simulink model "PMSM_SMO_SMC"  (R2022b)
settings: Solver=VariableStepAuto  StartTime=0.0  StopTime=4  FixedStep=1e-5  MaxStep=1E-5  RelTol=1e-4
values from neighbouring files (symbols this model uses):
  a_SMO = 0.6    [PMSM_SMO_SMC.m]
  Id_ref = 0    [PMSM_SMO_SMC.m]
  Ki_d = 100    [PMSM_SMO_SMC.m]
  Ki_q = 100    [PMSM_SMO_SMC.m]
  Kp_d = 0.1    [PMSM_SMO_SMC.m]
  Kp_q = 10    [PMSM_SMO_SMC.m]
  p = 4    [PMSM_SMO_SMC.m]
  Rs = 2.875    [PMSM_SMO_SMC.m]
  Ts = 1e-4    (= 0.0001)    [PMSM_SMO_SMC.m]
  Vdc = 310    [PMSM_SMO_SMC.m]
undefined symbols (not defined in the file or in its folder): sigbuilder_block
libraries: slpidlib x3, spsVoltageMeasurementLib x3, spsPermanentMagnetSynchronousMachineLib x2, mcbcontrolslib x2, spsAlphaBetaZerotodq0Lib x1, eeTransforms x1, spsDCVoltageSourceLib x1, spsTwoLevelConverterLib x1, spsThreePhaseVIMeasurementLib x1, spsSVPWMGenerator2LevelLib x1, spsdq0toAlphaBetaZeroLib x1, mcbsensorlessestimatorlib x1
settings Model: SimulationMode=accelerator  Creator=The MathWorks, Inc.  LastModifiedBy=DELL
settings DataIOCC: ExternalInput=[]  SaveFormat=Array  SaveOutput=off  SaveTime=off  ReturnWorkspaceOutputs=off  SignalLoggingName=sigsOut
settings OptimizationCC: BlockReduction=off  BooleanDataType=off  ExpressionDepthLimit=2147483647  InitFltsAndDblsToZero=on  EfficientMapNaN2IntZero=off  LifeSpan=inf
settings DebuggingCC: UnderspecifiedInitializationDetection=Classic  MergeDetectMultiDrivingBlocksExec=none  CheckExecutionContextPreStartOutputMsg=on  SignalResolutionControl=TryResolveAllWithWarning  MultiTaskDSMMsg=warning  MultiTaskCondExecSysMsg=none  SigSpecEnsureSampleTimeMsg=none  ParameterPrecisionLossMsg=none  FcnCallInpInsideContextMsg=warning  UnconnectedInputMsg=warning  UnconnectedOutputMsg=warning  UnconnectedLineMsg=warning  StateNameClashWarn=warning  SFUnexpectedBacktrackingDiag=warning  SFNoUnconditionalDefaultTransitionDiag=warning  SFExecutionAtInitializationDiag=none  SFMachineParentedDataDiag=warning  ArithmeticOperatorsInVariantConditions=warning
settings HardwareCC: ProdBitPerPointer=32  ProdBitPerSizeT=32  ProdBitPerPtrDiffT=32  ProdLargestAtomicFloat=None  ProdIntDivRoundTo=Undefined  ProdEndianess=Unspecified  ProdWordSize=32  ProdHWDeviceType=32-bit Generic  TargetUnknown=on
settings ModelReferenceCC: EnableRefExpFcnMdlSchedulingChecks=on  PropagateSignalLabelsOutOfModel=off
settings SFSimCC: SimUseLocalCustomCode=off  CustomCodeUndefinedFunction=UseInterfaceOnly
settings RTWCC: RTWUseLocalCustomCode=off
settings CodeAppCC: StateflowObjectComments=on
settings GRTTargetCC: TargetLangStandard=C89/C90 (ANSI)  CombineOutputUpdateFcns=off  GRTInterface=on
settings ConfigComp: CovMetricSettings=dw  CovSaveCumulativeToWorkspaceVar=on  CovSaveSingleToWorkspaceVar=on  CovExternalEMLEnable=off  CovSFcnEnable=off
settings SimscapeCC: SimscapeNormalizeSystem=off  SimscapeNominalValues={1, 'bar'; 1, 'cm^3/s'; 1, 'bar*kg/s'; 1, 'kJ/kg'; 1, 'kW'; }

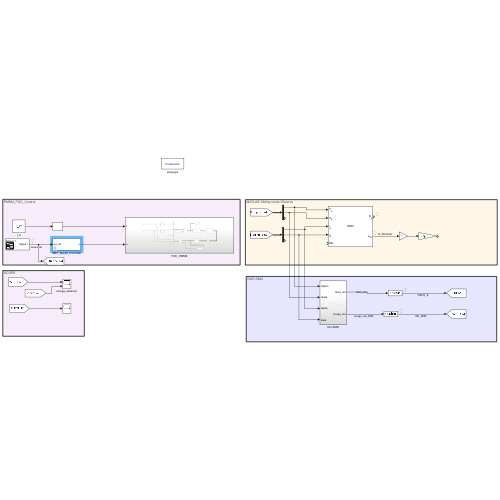
[thumbnail: Simulink's stored preview of the top-level diagram]
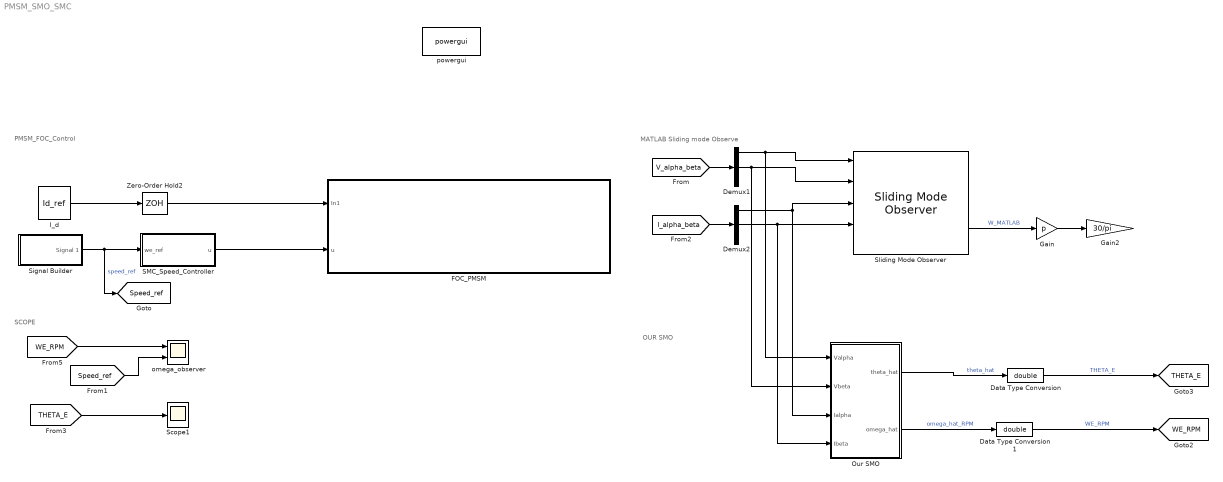
== system PMSM_SMO_SMC ==
  note: OUR SMO
  note: PMSM_FOC_Control
  note: MATLAB Sliding mode Observe
  note: SCOPE
  Data Type Conversion : DataTypeConversion  OutDataTypeStr=double  SaturateOnIntegerOverflow=off  RndMeth=Floor
  Data Type Conversion1 : DataTypeConversion  OutDataTypeStr=double  SaturateOnIntegerOverflow=off  RndMeth=Floor
  Demux1 : Demux  Outputs=3
  Demux2 : Demux  Outputs=3
  FOC_PMSM : Subsystem
  Gain : Gain  Gain=p
  Gain2 : Gain  Gain=30/pi  SaturateOnIntegerOverflow=on  OutDataTypeStr=Inherit: Same as input  ParamDataTypeStr=Inherit: Same as input
  I_d : Constant  Value=Id_ref
  Our SMO : Subsystem
  SMC_Speed_Controller : Subsystem  mask{TL=0.2, J=0.0008, B=0, p=4, lambda=0.175}
      mask prompts: TL "Torque Load"; J "Inetira"; B "Friction"; p "Pole"; lambda "flux linkage"
  Scope1 : Scope
  Signal Builder : Subsystem  Tag=STV Subsys  LoadFcn=sigbuilder_block('load');  StartFcn=sigbuilder_block('start');  StopFcn=sigbuilder_block('stop');  ClipboardFcn=sigbuilder_block('clipboard');  mask(Sigbuilder block){tuvar=[0:10]}
      mask help: Simulink:masks:SigbuilderBlock_MD
      mask init:
      | if ~strcmp(get_param(bdroot(gcbh),'SimulationStatus'),'stopped') tuvar = sigbuilder_block('maskInit'); end
      settings: CopyFcn=sigbuilder_block('copy');  DeleteFcn=sigbuilder_block('delete');  ModelCloseFcn=sigbuilder_block('modelClose');  PreSaveFcn=sigbuilder_block('preSave');  PauseFcn=sigbuilder_block('pause');  ContinueFcn=sigbuilder_block('continue');  NameChangeFcn=sigbuilder_block('namechange');  OpenFcn=sigbuilder_block('open',[437.6 199.2 550.4 400 ]);  CloseFcn=sigbuilder_block('close');
      mask Display: plot(0, 0, 100, 100,[2, 2, 32, 32, 2], [68, 8, 8, 68, 68],[32, 2], [38, 38], [32, 19, 2],[53, 60, 44], [32, 17, 17, 2],[16, 16, 31, 31]);txt = getActiveGroup(gcbh);text(2, 100, txt,'verticalAlignment', 'top');
  Sliding Mode Observer : mcbsensorlessestimatorlib/Sliding Mode Observer  InputUnit=SI unit  BlkSampleTime=1E-4  StatorResistance=StatorResistance  StatorInductance=StatorInductance  MaxApplicationSpeed=6000  PolePairs=PolePairs  MaxStatorVoltage=MaxStatorVoltage  MaxStatorCurrent=5  DisturbanceObserverGain=DisturbanceObserverGain  CurrentObserverGain=CurrentObserverGain  CutoffFreq=CutoffFreq  PositionUnit=Radians  PositionDataType=single  SpeedUnit=Radians/sec  PerUnitSpeed=6000  SpeedDataType=single
      settings: LibrarySourceBlock=mcblib/Sensorless Estimators/Sliding Mode Observer
  Zero-Order Hold2 : ZeroOrderHold  SampleTime=Ts
  omega_observer : Scope  NumInputPorts=2
  powergui : sps_lib/powergui  Priority=1  SimulationMode=Continuous  SampleTime=50e-6  frequency=60  Iterations=50  frequencyindice=0  Pbase=100e6  ErrMax=1e-4  UnitsV=kV  UnitsW=MW  buscounter=0  FunctionMessages=off  echomessages=off  EnableUseOfTLC=off  CurrentSourceSwitches=off  DisableSnubberDevices=off  DisableRonSwitches=off  DisableVfSwitches=off  DisplayEquations=off  AutomaticDiscreteSolvers=off  SolverType=Tustin/Backward Euler (TBE)  Interpol=off  ExternalGateDelay=off  methode=off  Ts=100  x0status=blocks  SPID=on  SwTol=0  HookPort=off  NonlinearTolerance=1e-4  nMaxIteration=100  ContinueOnMaxIteration=off  RestoreLinks=warning  ResistiveCurrentMeasurement=off  Frange=[0:2:500]  Ylog=off  Xlog=on  ShowGrid=off  save=off  variable=ZData  structure=0  ZoomFFT=off  StartTime=0.0  cycles=1  DisplayStyle=1  fundamental=60  FreqAxis=off  MaxFrequency=1000  frequencyindicesteady=1  RmsSteady=1  display=off
  tag scope: Speed_ref=global, THETA_E=global, WE_RPM=global
  wires:
  [V_alpha_beta] -> Demux1/1
  [I_alpha_beta] -> Demux2/1
  Gain/1 -> Gain2/1
  I_d/1 -> Zero-Order Hold2/1
  Zero-Order Hold2/1 -> FOC_PMSM/1(In1)
  Sliding Mode Observer/2 -> Gain/1  "W_MATLAB"
  Demux1/1 -> Our SMO/1(Valpha), Sliding Mode Observer/1
  Demux1/2 -> Our SMO/2(Vbeta), Sliding Mode Observer/2
  Demux2/1 -> Our SMO/3(Ialpha), Sliding Mode Observer/3
  Demux2/2 -> Our SMO/4(Ibeta), Sliding Mode Observer/4
  Our SMO/2(omega_hat) -> Data Type Conversion1/1  "omega_hat_RPM"
  Data Type Conversion/1 -> [THETA_E]  "THETA_E"
  Data Type Conversion1/1 -> [WE_RPM]  "WE_RPM"
  SMC_Speed_Controller/1(u) -> FOC_PMSM/2(u)
  Our SMO/1(theta_hat) -> Data Type Conversion/1  "theta_hat"
  Signal Builder/1(Signal 1) -> [Speed_ref], SMC_Speed_Controller/1(we_ref)  "speed_ref"
  [WE_RPM] -> omega_observer/1
  [THETA_E] -> Scope1/1
  [Speed_ref] -> omega_observer/2

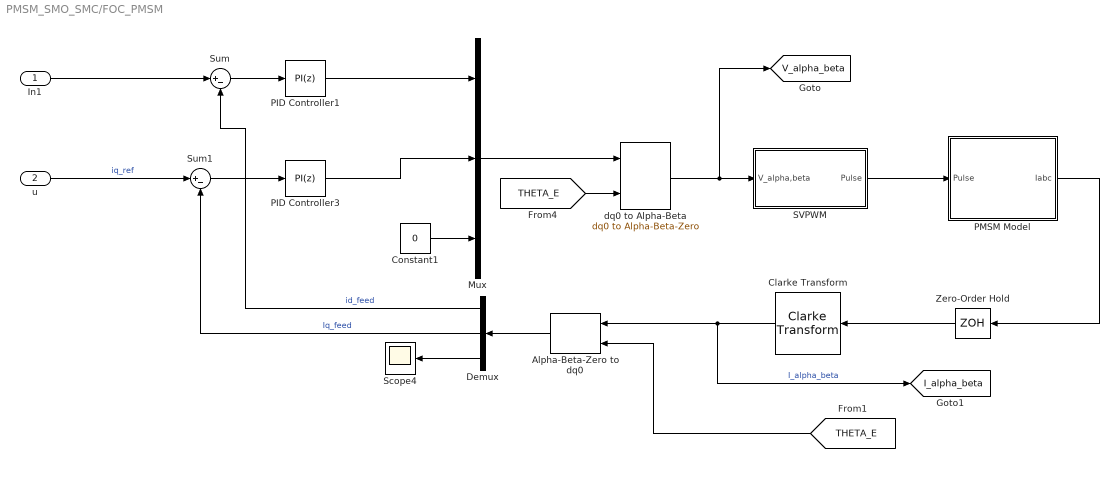
== system PMSM_SMO_SMC/FOC_PMSM ==
  In1 : Inport
  u : Inport  Port=2
  Alpha-Beta-Zero to dq0 : spsAlphaBetaZerotodq0Lib/Alpha-Beta-Zero to dq0  Alignment=Aligned with phase A axis
  Clarke Transform : eeTransforms/Clarke Transform  PowerInvariant=off
      settings: LibrarySourceBlock=|
      | ee_sl_lib/Mathematical
      | Transforms/Clarke Transform
  Constant1 : Constant  Value=0
  Demux : Demux  Outputs=3
  Mux : Mux  Inputs=3
  PID Controller1 : slpidlib/PID Controller  Controller=PI  Form=Parallel  TimeDomain=Discrete-time  UseExternalTs=off  SampleTime=1E-4  IntegratorMethod=Forward Euler  FilterMethod=Forward Euler  ControllerParametersSource=internal  P=Kp_d  I=Ki_d  UseKiTs=off  D=0  N=100  UseFilter=on  TunerSelectOption=Transfer Function Based (PID Tuner App)  InitialConditionSource=internal  InitialConditionForIntegrator=0  InitialConditionForFilter=0  DifferentiatorICPrevScaledInput=0  ExternalReset=none  TrackingMode=off  Kt=1  LimitOutput=off  SatLimitsSource=internal  UpperSaturationLimit=inf  LowerSaturationLimit=-inf  LinearizeAsGain=on  AntiWindupMode=none  Kb=1  LimitIntegrator=off  UpperIntegratorSaturationLimit=inf  LowerIntegratorSaturationLimit=-inf  POutMin=[]  POutMax=[]  IOutMin=[]  IOutMax=[]  DOutMin=[]  DOutMax=[]  NOutMin=[]  NOutMax=[]  SumOutMin=[]  SumOutMax=[]  SaturationOutMin=[]  SaturationOutMax=[]  PParamMin=[]  PParamMax=[]  IParamMin=[]  IParamMax=[]  DParamMin=[]  DParamMax=[]  NParamMin=[]  NParamMax=[]  KbParamMin=[]  KbParamMax=[]  KtParamMin=[]  KtParamMax=[]  KbOutMin=[]  KbOutMax=[]  KtOutMin=[]  KtOutMax=[]  IntegratorOutMin=[]  IntegratorOutMax=[]  FilterOutMin=[]  FilterOutMax=[]  SumI1OutMin=[]  SumI1OutMax=[]  SumI2OutMin=[]  SumI2OutMax=[]  SumI3OutMin=[]  SumI3OutMax=[]  SumI4OutMin=[]  SumI4OutMax=[]  SumDOutMin=[]  SumDOutMax=[]  DifferentiatorOutMin=[]  DifferentiatorOutMax=[]  FilterDiffOutCoefMin=[]  FilterDiffOutCoefMax=[]  ReciprocalOutMin=[]  ReciprocalOutMax=[]  SumDenOutMin=[]  SumDenOutMax=[]  SumNumOutMin=[]  SumNumOutMax=[]  DivideOutMin=[]  DivideOutMax=[]  UdiffTsProdOutMin=[]  UdiffTsProdOutMax=[]  NTsProdOutMin=[]  NTsProdOutMax=[]  UintegralTsProdOutMin=[]  UintegralTsProdOutMax=[]  UngainTsProdOutMin=[]  UngainTsProdOutMax=[]  ClampingZeroOutDataTypeStr=Inherit: Inherit via back propagation  ClampingZeroOutMin=[]  ClampingZeroOutMax=[]  FilterDenConstantOutDataTypeStr=Inherit: Inherit via back propagation  FilterDenConstantOutMin=[]  FilterDenConstantOutMax=[]  PCopyOutDataTypeStr=Inherit: Inherit via back propagation  PCopyOutMin=[]  PCopyOutMax=[]  NCopyOutDataTypeStr=Inherit: Inherit via back propagation  NCopyOutMin=[]  NCopyOutMax=[]  IntegratorContinuousStateAttributes=''  IntegratorStateMustResolveToSignalObject=off  IntegratorRTWStateStorageClass=Auto  FilterContinuousStateAttributes=''  FilterStateMustResolveToSignalObject=off  FilterRTWStateStorageClass=Auto  ParallelPVariant=InternalParameters  IdealPVariant=Disabled  IVariant=InternalParameters  DVariant=Disabled  IntegratorVariant=Discrete  SatVariant=Disabled  AWVariant=Passthrough  PCopyVariant=Disabled  TRVariant=Disabled  FdbkBlocksVariant=Forward  IdealPFdbkVariant=Disabled  SatFdbkVariant=Disabled  DerivativeFilterVariant=Disabled  NVariant=Disabled  NCopyVariant=Disabled_SignalSpec  FilterICVariant=Disabled  IntegratorICVariant=InternalICs  ExternalResetVariant=Disabled  TRSumVariant=Passthrough  SumFdbkVariant=Disabled  SumVariant=Sum_PI  TsampFilterVariant=InternalTs  TsampNgainVariant=Passthrough  TsampIntegralVariant=Passthrough  ExternalSaturationOutDataTypeStr=Inherit: Same as second input
  PID Controller3 : slpidlib/PID Controller  Controller=PI  Form=Parallel  TimeDomain=Discrete-time  UseExternalTs=off  SampleTime=1E-4  IntegratorMethod=Forward Euler  FilterMethod=Forward Euler  ControllerParametersSource=internal  P=Kp_q  I=Ki_q  UseKiTs=off  D=0  N=100  UseFilter=on  TunerSelectOption=Transfer Function Based (PID Tuner App)  InitialConditionSource=internal  InitialConditionForIntegrator=0  InitialConditionForFilter=0  DifferentiatorICPrevScaledInput=0  ExternalReset=none  TrackingMode=off  Kt=1  LimitOutput=off  SatLimitsSource=internal  UpperSaturationLimit=inf  LowerSaturationLimit=-inf  LinearizeAsGain=on  AntiWindupMode=none  Kb=1  LimitIntegrator=off  UpperIntegratorSaturationLimit=inf  LowerIntegratorSaturationLimit=-inf  POutMin=[]  POutMax=[]  IOutMin=[]  IOutMax=[]  DOutMin=[]  DOutMax=[]  NOutMin=[]  NOutMax=[]  SumOutMin=[]  SumOutMax=[]  SaturationOutMin=[]  SaturationOutMax=[]  PParamMin=[]  PParamMax=[]  IParamMin=[]  IParamMax=[]  DParamMin=[]  DParamMax=[]  NParamMin=[]  NParamMax=[]  KbParamMin=[]  KbParamMax=[]  KtParamMin=[]  KtParamMax=[]  KbOutMin=[]  KbOutMax=[]  KtOutMin=[]  KtOutMax=[]  IntegratorOutMin=[]  IntegratorOutMax=[]  FilterOutMin=[]  FilterOutMax=[]  SumI1OutMin=[]  SumI1OutMax=[]  SumI2OutMin=[]  SumI2OutMax=[]  SumI3OutMin=[]  SumI3OutMax=[]  SumI4OutMin=[]  SumI4OutMax=[]  SumDOutMin=[]  SumDOutMax=[]  DifferentiatorOutMin=[]  DifferentiatorOutMax=[]  FilterDiffOutCoefMin=[]  FilterDiffOutCoefMax=[]  ReciprocalOutMin=[]  ReciprocalOutMax=[]  SumDenOutMin=[]  SumDenOutMax=[]  SumNumOutMin=[]  SumNumOutMax=[]  DivideOutMin=[]  DivideOutMax=[]  UdiffTsProdOutMin=[]  UdiffTsProdOutMax=[]  NTsProdOutMin=[]  NTsProdOutMax=[]  UintegralTsProdOutMin=[]  UintegralTsProdOutMax=[]  UngainTsProdOutMin=[]  UngainTsProdOutMax=[]  ClampingZeroOutDataTypeStr=Inherit: Inherit via back propagation  ClampingZeroOutMin=[]  ClampingZeroOutMax=[]  FilterDenConstantOutDataTypeStr=Inherit: Inherit via back propagation  FilterDenConstantOutMin=[]  FilterDenConstantOutMax=[]  PCopyOutDataTypeStr=Inherit: Inherit via back propagation  PCopyOutMin=[]  PCopyOutMax=[]  NCopyOutDataTypeStr=Inherit: Inherit via back propagation  NCopyOutMin=[]  NCopyOutMax=[]  IntegratorContinuousStateAttributes=''  IntegratorStateMustResolveToSignalObject=off  IntegratorRTWStateStorageClass=Auto  FilterContinuousStateAttributes=''  FilterStateMustResolveToSignalObject=off  FilterRTWStateStorageClass=Auto  ParallelPVariant=InternalParameters  IdealPVariant=Disabled  IVariant=InternalParameters  DVariant=Disabled  IntegratorVariant=Discrete  SatVariant=Disabled  AWVariant=Passthrough  PCopyVariant=Disabled  TRVariant=Disabled  FdbkBlocksVariant=Forward  IdealPFdbkVariant=Disabled  SatFdbkVariant=Disabled  DerivativeFilterVariant=Disabled  NVariant=Disabled  NCopyVariant=Disabled_SignalSpec  FilterICVariant=Disabled  IntegratorICVariant=InternalICs  ExternalResetVariant=Disabled  TRSumVariant=Passthrough  SumFdbkVariant=Disabled  SumVariant=Sum_PI  TsampFilterVariant=InternalTs  TsampNgainVariant=Passthrough  TsampIntegralVariant=Passthrough  ExternalSaturationOutDataTypeStr=Inherit: Same as second input
  PMSM Model : Subsystem
  SVPWM : Subsystem
  Scope4 : Scope
  Sum : Sum  Inputs=|+-
  Sum1 : Sum  Inputs=|+-
  Zero-Order Hold : ZeroOrderHold  SampleTime=Ts
  dq0 to Alpha-Beta : spsdq0toAlphaBetaZeroLib/dq0 to Alpha-Beta-Zero  Alignment=Aligned with phase A axis
  tag scope: I_alpha_beta=global, V_alpha_beta=global
  wires:
  [THETA_E] -> Alpha-Beta-Zero to dq0/2
  Clarke Transform/1 -> [I_alpha_beta], Alpha-Beta-Zero to dq0/1  "I_alpha_beta"
  PMSM Model/1(Iabc) -> Zero-Order Hold/1
  Mux/1 -> dq0 to Alpha-Beta/1
  u/1 -> Sum1/1  "iq_ref"
  Sum1/1 -> PID Controller3/1
  SVPWM/1(Pulse) -> PMSM Model/1(Pulse)
  dq0 to Alpha-Beta/1 -> [V_alpha_beta], SVPWM/1(V_alpha,beta)
  Demux/1 -> Sum/2  "id_feed"
  Constant1/1 -> Mux/3
  Demux/3 -> Scope4/1
  [THETA_E] -> dq0 to Alpha-Beta/2
  Sum/1 -> PID Controller1/1
  Demux/2 -> Sum1/2  "Iq_feed"
  Alpha-Beta-Zero to dq0/1 -> Demux/1
  In1/1 -> Sum/1
  Zero-Order Hold/1 -> Clarke Transform/1
  PID Controller1/1 -> Mux/1
  PID Controller3/1 -> Mux/2

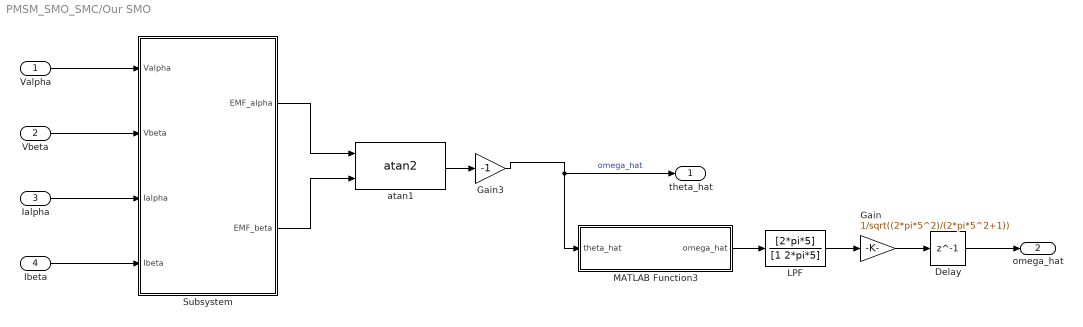
== system PMSM_SMO_SMC/Our SMO ==
  Valpha : Inport
  Vbeta : Inport  Port=2
  Ialpha : Inport  Port=3
  Ibeta : Inport  Port=4
  Delay : Delay  DelayLength=1
  Gain : Gain  Gain=1/sqrt((2*pi*5^2)/(2*pi*5^2+1))
  Gain3 : Gain  Gain=-1
  LPF : TransferFcn  Numerator=[2*pi*5]  Denominator=[1 2*pi*5]
  MATLAB Function3 : MATLAB Function  TreatAsAtomicUnit=on
  Subsystem : Subsystem
  atan1 : mcbcontrolslib/atan2  outputUnit=Radians
  theta_hat : Outport
  omega_hat : Outport  Port=2
  wires:
  Valpha/1 -> Subsystem/1(Valpha)
  Vbeta/1 -> Subsystem/2(Vbeta)
  Ialpha/1 -> Subsystem/3(Ialpha)
  Ibeta/1 -> Subsystem/4(Ibeta)
  atan1/1 -> Gain3/1
  MATLAB Function3/1(omega_hat) -> LPF/1
  LPF/1 -> Gain/1
  Gain3/1 -> theta_hat/1, MATLAB Function3/1(theta_hat)  "omega_hat"
  Subsystem/1(EMF_alpha) -> atan1/1
  Subsystem/2(EMF_beta) -> atan1/2
  Delay/1 -> omega_hat/1
  Gain/1 -> Delay/1

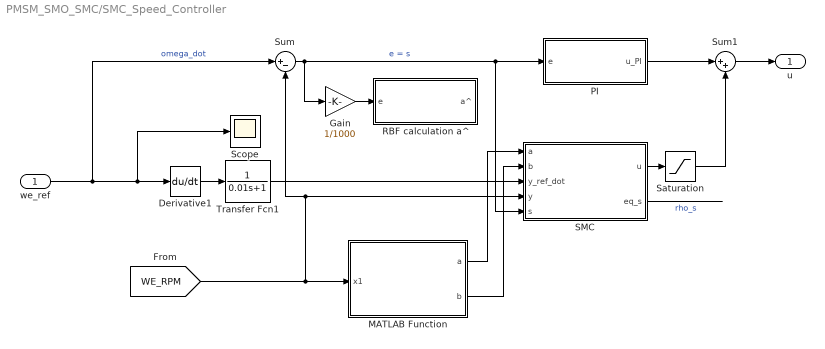
== system PMSM_SMO_SMC/SMC_Speed_Controller ==
  we_ref : Inport
  Derivative1 : Derivative
  Gain : Gain  Gain=1/1000
  MATLAB Function : MATLAB Function  TreatAsAtomicUnit=on
  PI : Subsystem
  RBF calculation a^ : Subsystem
  SMC : MATLAB Function  TreatAsAtomicUnit=on
  Saturation : Saturate  UpperLimit=3  LowerLimit=-3
  Scope : Scope
  Sum : Sum  Inputs=|+-
  Sum1 : Sum  Inputs=|++
  Transfer Fcn1 : TransferFcn  Denominator=[0.01 1]
  u : Outport
  wires:
  [WE_RPM] -> Sum/2, SMC/4(y), MATLAB Function/1(x1)
  we_ref/1 -> Derivative1/1, Scope/1, Sum/1  "omega_dot"
  MATLAB Function/2(b) -> SMC/2(b)
  Sum/1 -> Gain/1, PI/1(e), SMC/5(s)  "e = s"
  SMC/1(u) -> Saturation/1
  SMC/2(eq_s) -> ?  "rho_s"
  Gain/1 -> RBF calculation a^/1(e)
  MATLAB Function/1(a) -> SMC/1(a)
  Derivative1/1 -> Transfer Fcn1/1
  Transfer Fcn1/1 -> SMC/3(y_ref_dot)
  PI/1(u_PI) -> Sum1/1
  Saturation/1 -> Sum1/2
  Sum1/1 -> u/1

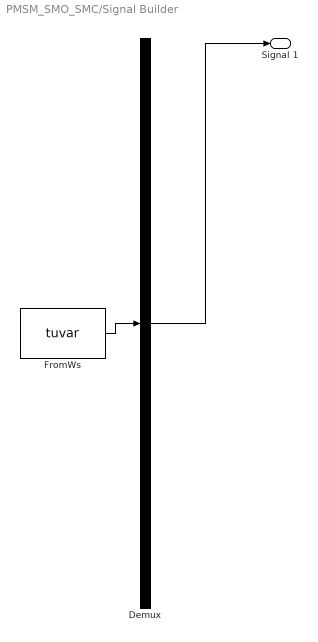
== system PMSM_SMO_SMC/Signal Builder ==
  Demux : Demux  Tag=STV Demux  Outputs=1
      settings: DisplayOption=none
  FromWs : FromWorkspace  Tag=STV FromWs  VariableName=tuvar
      SigBuilderData=|
      | common.afterFinalStr = 'Extrapolate'
      | common.sampleTime = 0
      | dataSet.timeRange = [0 10]
      | dataSet.name = 'Group 1'
      | sbobj.Groups.Name = 'Group 1'
      | sbobj.Groups.Signals.Name = 'Signal 1'
      | sbobj.Groups.Signals.XData = [0 4 4 6 6 8.04 8.04 10]
      | sbobj.Groups.Signals.YData = [1000 1000 200 200 1000 1000 600 600]
  Signal 1 : Outport  Tag=STV Outport
  wires:
  Demux/1 -> Signal 1/1
  FromWs/1 -> Demux/1

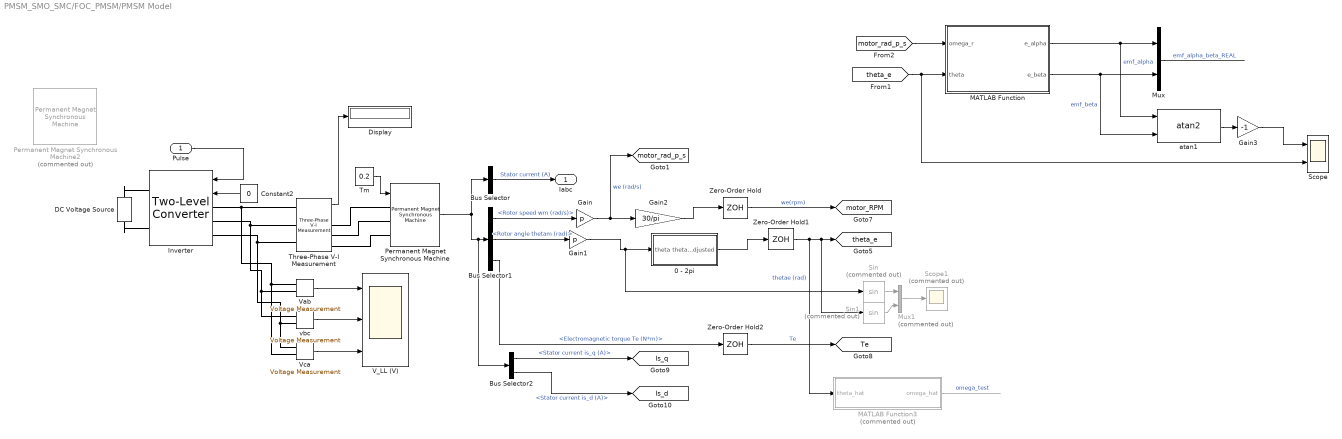
== system PMSM_SMO_SMC/FOC_PMSM/PMSM Model ==
  Pulse : Inport
  0 - 2pi : MATLAB Function  TreatAsAtomicUnit=on
  Bus Selector : BusSelector  OutputSignals=Stator current is_a (A),Stator current is_b (A),Stator current is_c (A)  OutputAsBus=on
  Bus Selector1 : BusSelector  OutputSignals=Rotor speed wm (rad/s),Rotor angle thetam (rad),Electromagnetic torque Te (N*m)
  Bus Selector2 : BusSelector  OutputSignals=Stator current is_q (A),Stator current is_d (A)
  Constant2 : Constant  Value=0
  "DC Voltage Source  " : spsDCVoltageSourceLib/DC Voltage Source  Amplitude=Vdc  Measurements=Voltage
  Display : Display
  Gain : Gain  Gain=p  SaturateOnIntegerOverflow=on  OutDataTypeStr=Inherit: Same as input  ParamDataTypeStr=Inherit: Same as input
  Gain1 : Gain  Gain=p  SaturateOnIntegerOverflow=on  OutDataTypeStr=Inherit: Same as input  ParamDataTypeStr=Inherit: Same as input
  Gain2 : Gain  Gain=30/pi  SaturateOnIntegerOverflow=on  OutDataTypeStr=Inherit: Same as input  ParamDataTypeStr=Inherit: Same as input
  Gain3 : Gain  Gain=-1
  Inverter : spsTwoLevelConverterLib/Two-Level Converter  ModelType=Switching devices  Ron=1e-3  Rs=1e6  Cs=inf  Vforward=[0,0]  Ron_Diode=1e-3  Rs_Diode=1e6  Cs_Diode=inf  Vf_Diode=1e-3  Rs_CurrentSource=inf  Ron_ACsource=1e-3
      settings: LibrarySourceBlock=sps_lib/Power Electronics/Two-Level Converter
  MATLAB Function : MATLAB Function  TreatAsAtomicUnit=on
  MATLAB Function3 : MATLAB Function  Commented=on  TreatAsAtomicUnit=on
  Mux : Mux  Inputs=2
  Mux1 : Mux  Commented=on  Inputs=2
  Permanent Magnet Synchronous Machine : spsPermanentMagnetSynchronousMachineLib/Permanent Magnet Synchronous Machine  NbPhases=3  FluxDistribution=Sinusoidal  RotorType=Round  MechanicalLoad=Torque Tm  PresetModel=No  ShowDetailedParameters=on  MeasurementBus=off  Resistance=Rs  Inductance=8.5e-3  dqInductances=[8.5e-3,8.5e-3]  La=Ls  MachineConstant=Flux linkage established by magnets (V.s)  Flux=lambda  VoltageCst=126.966  TorqueCst=1.05  Flat=120  Mechanical=[0.0008 1.349e-05 p 0]  PolePairs=4  InitialConditions=[0,0,0,0]  InitialConditions5ph=[0 0 0 0 0 0]  RefAngle=Aligned with phase A axis (original Park)  IterativeDiscreteModel=Trapezoidal non iterative  TsBlock=-1  TsPowergui=0
  Permanent Magnet Synchronous Machine2 : spsPermanentMagnetSynchronousMachineLib/Permanent Magnet Synchronous Machine  Commented=on  NbPhases=3  FluxDistribution=Sinusoidal  RotorType=Round  MechanicalLoad=Torque Tm  PresetModel=No  ShowDetailedParameters=on  MeasurementBus=off  Resistance=2.87  Inductance=8.5e-3  dqInductances=[8.5e-3,8.5e-3]  La=8.5*1e-3  MachineConstant=Flux linkage established by magnets (V.s)  Flux=0.175  VoltageCst=63.483  TorqueCst=0.525  Flat=120  Mechanical=[0.0008 1.349e-05 2 0]  PolePairs=2  InitialConditions=[0,0,0,0]  InitialConditions5ph=[0 0 0 0 0 0]  RefAngle=Aligned with phase A axis (original Park)  IterativeDiscreteModel=Trapezoidal non iterative  TsBlock=-1  TsPowergui=0
  Scope : Scope  NumInputPorts=2
  Scope1 : Scope  Commented=on
  Sin : Trigonometry  Commented=on
  Sin1 : Trigonometry  Commented=on
  Three-Phase V-I Measurement : spsThreePhaseVIMeasurementLib/Three-Phase V-I Measurement  VoltageMeasurement=phase-to-phase  SetLabelV=off  LabelV=Vabc  Vpu=off  VpuLL=off  CurrentMeasurement=yes  SetLabelI=off  LabelI=Iabc  Ipu=off  Pbase=100e6  Vbase=500e3  OutputType=Complex  PhasorSimulation=off  PSBequivalent=0
  Tm : Constant  Value=0.2
  V_LL (V) : Scope  NumInputPorts=3
  Vab : spsVoltageMeasurementLib/Voltage Measurement  Tag=PoWeRsYsTeMmEaSuReMeNt  PhasorSimulation=off  OutputType=Magnitude  PSBequivalent=0
  Vca : spsVoltageMeasurementLib/Voltage Measurement  Tag=PoWeRsYsTeMmEaSuReMeNt  PhasorSimulation=off  OutputType=Magnitude  PSBequivalent=0
  Zero-Order Hold : ZeroOrderHold  SampleTime=Ts
  Zero-Order Hold1 : ZeroOrderHold  SampleTime=Ts
  Zero-Order Hold2 : ZeroOrderHold  SampleTime=Ts
  atan1 : mcbcontrolslib/atan2  outputUnit=Radians
  vbc : spsVoltageMeasurementLib/Voltage Measurement  Tag=PoWeRsYsTeMmEaSuReMeNt  PhasorSimulation=off  OutputType=Magnitude  PSBequivalent=0
  Iabc : Outport
  tag scope: Is_d=global, Is_q=global, Te=global, motor_RPM=global, motor_rad_p_s=global, theta_e=global
  wires:
  Bus Selector1/1 -> Gain/1  "<Rotor speed wm (rad/s)>"
  Gain/1 -> [motor_rad_p_s], Gain2/1  "we (rad/s)"
  Permanent Magnet Synchronous Machine/1 -> Bus Selector/1, Bus Selector2/1, Bus Selector1/1
  Bus Selector1/2 -> Gain1/1  "<Rotor angle thetam (rad)>"
  Gain2/1 -> Zero-Order Hold/1
  Bus Selector/1 -> Iabc/1  "Stator current (A)"
  Bus Selector2/1 -> [Is_q]  "<Stator current is_q (A)>"
  Bus Selector1/3 -> Zero-Order Hold2/1  "<Electromagnetic torque Te (N*m)>"
  Bus Selector2/2 -> [Is_d]  "<Stator current is_d (A)>"
  Tm/1 -> Permanent Magnet Synchronous Machine/1
  vbc/1 -> V_LL (V)/2
  Vca/1 -> V_LL (V)/3
  Vab/1 -> V_LL (V)/1
  Pulse/1 -> Inverter/1
  Constant2/1 -> Inverter/2
  Zero-Order Hold/1 -> [motor_RPM]  "we(rpm)"
  Zero-Order Hold1/1 -> MATLAB Function3/1(theta_hat), Sin1/1, [theta_e]  "thetae (rad)"
  Zero-Order Hold2/1 -> [Te]  "Te"
  Three-Phase V-I Measurement/1 -> Display/1
  0 - 2pi/1(theta_adjusted) -> Zero-Order Hold1/1
  [motor_rad_p_s] -> MATLAB Function/1(omega_r)
  [theta_e] -> Scope/2, MATLAB Function/2(theta)
  MATLAB Function/1(e_alpha) -> atan1/1, Mux/1  "emf_alpha"
  MATLAB Function/2(e_beta) -> atan1/2, Mux/2  "emf_beta"
  Mux/1 -> ?  "emf_alpha_beta_REAL"
  atan1/1 -> Gain3/1
  Gain3/1 -> Scope/1
  MATLAB Function3/1(omega_hat) -> ?  "omega_test"
  Gain1/1 -> Sin/1, 0 - 2pi/1(theta)
  Sin/1 -> Mux1/1
  Sin1/1 -> Mux1/2
  Mux1/1 -> Scope1/1
  connections:
  vbc/LConn1 -- Inverter/LConn2 -- Three-Phase V-I Measurement/LConn2 -- Vab/LConn2
  vbc/LConn2 -- Inverter/LConn3 -- Three-Phase V-I Measurement/LConn3 -- Vca/LConn1
  Vab/LConn1 -- Three-Phase V-I Measurement/LConn1 -- Inverter/LConn1 -- Vca/LConn2
  "DC Voltage Source  "/RConn1 -- Inverter/RConn1
  "DC Voltage Source  "/LConn1 -- Inverter/RConn2
  Three-Phase V-I Measurement/RConn1 -- Permanent Magnet Synchronous Machine/LConn1
  Three-Phase V-I Measurement/RConn2 -- Permanent Magnet Synchronous Machine/LConn2
  Three-Phase V-I Measurement/RConn3 -- Permanent Magnet Synchronous Machine/LConn3

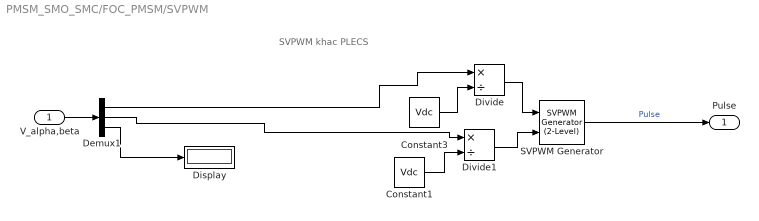
== system PMSM_SMO_SMC/FOC_PMSM/SVPWM ==
  note: SVPWM khac PLECS
  V_alpha,beta : Inport
  Constant1 : Constant  Value=Vdc
  Constant3 : Constant  Value=Vdc
  Demux1 : Demux  Outputs=3
  Display : Display
  Divide : Product  Inputs=*/
  Divide1 : Product  Inputs=*/
  SVPWM Generator : spsSVPWMGenerator2LevelLib/SVPWM Generator (2-Level)  InputType=alpha-beta components  SwitchingPattern=Pattern #1  Fc=10000  ParUref=[0.8 -30 50]  Ts=0
  Pulse : Outport
  wires:
  Demux1/2 -> Divide1/1
  Demux1/3 -> Display/1
  Demux1/1 -> Divide/1
  Divide/1 -> SVPWM Generator/1
  V_alpha,beta/1 -> Demux1/1
  Constant3/1 -> Divide/2
  SVPWM Generator/1 -> Pulse/1  "Pulse"
  Constant1/1 -> Divide1/2
  Divide1/1 -> SVPWM Generator/2

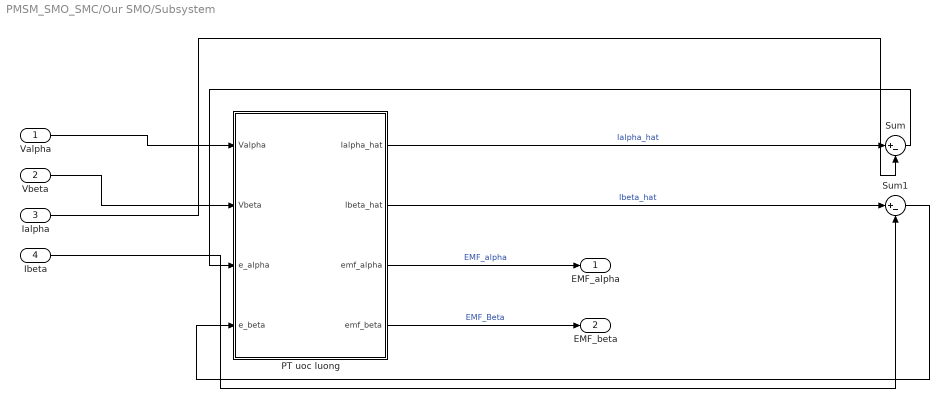
== system PMSM_SMO_SMC/Our SMO/Subsystem ==
  Valpha : Inport
  Vbeta : Inport  Port=2
  Ialpha : Inport  Port=3
  Ibeta : Inport  Port=4
  PT uoc luong : Subsystem
  Sum : Sum  Inputs=|+-
  Sum1 : Sum  Inputs=|+-
  EMF_alpha : Outport
  EMF_beta : Outport  Port=2
  wires:
  PT uoc luong/2(Ibeta_hat) -> Sum1/1  "Ibeta_hat"
  Sum1/1 -> PT uoc luong/4(e_beta)
  PT uoc luong/1(Ialpha_hat) -> Sum/1  "Ialpha_hat"
  Ibeta/1 -> Sum1/2
  Ialpha/1 -> Sum/2
  Sum/1 -> PT uoc luong/3(e_alpha)
  Valpha/1 -> PT uoc luong/1(Valpha)
  Vbeta/1 -> PT uoc luong/2(Vbeta)
  PT uoc luong/3(emf_alpha) -> EMF_alpha/1  "EMF_alpha"
  PT uoc luong/4(emf_beta) -> EMF_beta/1  "EMF_Beta"

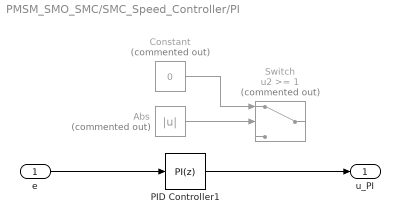
== system PMSM_SMO_SMC/SMC_Speed_Controller/PI ==
  e : Inport
  Abs : Abs  Commented=on  SaturateOnIntegerOverflow=off
  Constant : Constant  Commented=on  Value=0
  PID Controller1 : slpidlib/PID Controller  Controller=PI  Form=Parallel  TimeDomain=Discrete-time  UseExternalTs=off  SampleTime=1E-4  IntegratorMethod=Forward Euler  FilterMethod=Forward Euler  ControllerParametersSource=internal  P=0  I=0.1  UseKiTs=off  D=0  N=100  UseFilter=on  TunerSelectOption=Transfer Function Based (PID Tuner App)  InitialConditionSource=internal  InitialConditionForIntegrator=0  InitialConditionForFilter=0  DifferentiatorICPrevScaledInput=0  ExternalReset=none  TrackingMode=off  Kt=1  LimitOutput=off  SatLimitsSource=internal  UpperSaturationLimit=inf  LowerSaturationLimit=-inf  LinearizeAsGain=on  AntiWindupMode=none  Kb=1  LimitIntegrator=off  UpperIntegratorSaturationLimit=inf  LowerIntegratorSaturationLimit=-inf  POutMin=[]  POutMax=[]  IOutMin=[]  IOutMax=[]  DOutMin=[]  DOutMax=[]  NOutMin=[]  NOutMax=[]  SumOutMin=[]  SumOutMax=[]  SaturationOutMin=[]  SaturationOutMax=[]  PParamMin=[]  PParamMax=[]  IParamMin=[]  IParamMax=[]  DParamMin=[]  DParamMax=[]  NParamMin=[]  NParamMax=[]  KbParamMin=[]  KbParamMax=[]  KtParamMin=[]  KtParamMax=[]  KbOutMin=[]  KbOutMax=[]  KtOutMin=[]  KtOutMax=[]  IntegratorOutMin=[]  IntegratorOutMax=[]  FilterOutMin=[]  FilterOutMax=[]  SumI1OutMin=[]  SumI1OutMax=[]  SumI2OutMin=[]  SumI2OutMax=[]  SumI3OutMin=[]  SumI3OutMax=[]  SumI4OutMin=[]  SumI4OutMax=[]  SumDOutMin=[]  SumDOutMax=[]  DifferentiatorOutMin=[]  DifferentiatorOutMax=[]  FilterDiffOutCoefMin=[]  FilterDiffOutCoefMax=[]  ReciprocalOutMin=[]  ReciprocalOutMax=[]  SumDenOutMin=[]  SumDenOutMax=[]  SumNumOutMin=[]  SumNumOutMax=[]  DivideOutMin=[]  DivideOutMax=[]  UdiffTsProdOutMin=[]  UdiffTsProdOutMax=[]  NTsProdOutMin=[]  NTsProdOutMax=[]  UintegralTsProdOutMin=[]  UintegralTsProdOutMax=[]  UngainTsProdOutMin=[]  UngainTsProdOutMax=[]  ClampingZeroOutDataTypeStr=Inherit: Inherit via back propagation  ClampingZeroOutMin=[]  ClampingZeroOutMax=[]  FilterDenConstantOutDataTypeStr=Inherit: Inherit via back propagation  FilterDenConstantOutMin=[]  FilterDenConstantOutMax=[]  PCopyOutDataTypeStr=Inherit: Inherit via back propagation  PCopyOutMin=[]  PCopyOutMax=[]  NCopyOutDataTypeStr=Inherit: Inherit via back propagation  NCopyOutMin=[]  NCopyOutMax=[]  IntegratorContinuousStateAttributes=''  IntegratorStateMustResolveToSignalObject=off  IntegratorRTWStateStorageClass=Auto  FilterContinuousStateAttributes=''  FilterStateMustResolveToSignalObject=off  FilterRTWStateStorageClass=Auto  ParallelPVariant=InternalParameters  IdealPVariant=Disabled  IVariant=InternalParameters  DVariant=Disabled  IntegratorVariant=Discrete  SatVariant=Disabled  AWVariant=Passthrough  PCopyVariant=Disabled  TRVariant=Disabled  FdbkBlocksVariant=Forward  IdealPFdbkVariant=Disabled  SatFdbkVariant=Disabled  DerivativeFilterVariant=Disabled  NVariant=Disabled  NCopyVariant=Disabled_SignalSpec  FilterICVariant=Disabled  IntegratorICVariant=InternalICs  ExternalResetVariant=Disabled  TRSumVariant=Passthrough  SumFdbkVariant=Disabled  SumVariant=Sum_PI  TsampFilterVariant=InternalTs  TsampNgainVariant=Passthrough  TsampIntegralVariant=Passthrough  ExternalSaturationOutDataTypeStr=Inherit: Same as second input
  Switch : Switch  Commented=on  Threshold=1  SaturateOnIntegerOverflow=off  InputSameDT=off
  u_PI : Outport
  wires:
  e/1 -> PID Controller1/1
  PID Controller1/1 -> u_PI/1
  Constant/1 -> Switch/1
  Abs/1 -> Switch/2
  ? -> Abs/1

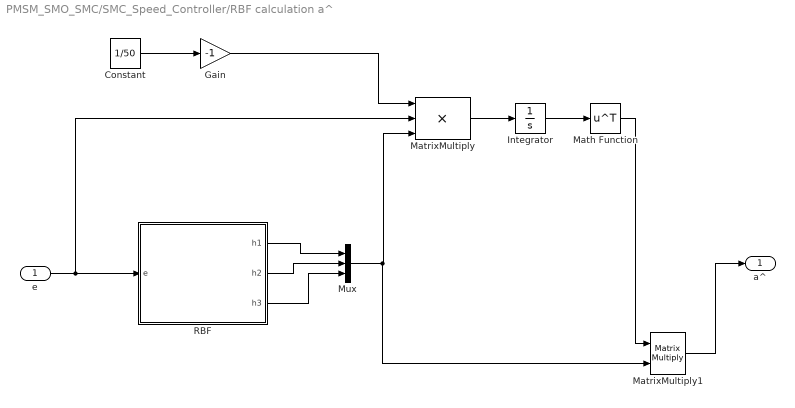
== system PMSM_SMO_SMC/SMC_Speed_Controller/RBF calculation a^ ==
  e : Inport
  Constant : Constant  Value=1/50
  Gain : Gain  Gain=-1
  Integrator : Integrator
  Math Function : Math  Operator=transpose
  MatrixMultiply : Product  Inputs=3
  MatrixMultiply1 : Product  Multiplication=Matrix(*)
  Mux : Mux  Inputs=3
  RBF : MATLAB Function  TreatAsAtomicUnit=on
  a^ : Outport
  wires:
  e/1 -> MatrixMultiply/2, RBF/1(e)
  RBF/1(h1) -> Mux/1
  RBF/2(h2) -> Mux/2
  RBF/3(h3) -> Mux/3
  Mux/1 -> MatrixMultiply1/2, MatrixMultiply/3
  Constant/1 -> Gain/1
  Gain/1 -> MatrixMultiply/1
  MatrixMultiply/1 -> Integrator/1
  Integrator/1 -> Math Function/1
  Math Function/1 -> MatrixMultiply1/1
  MatrixMultiply1/1 -> a^/1

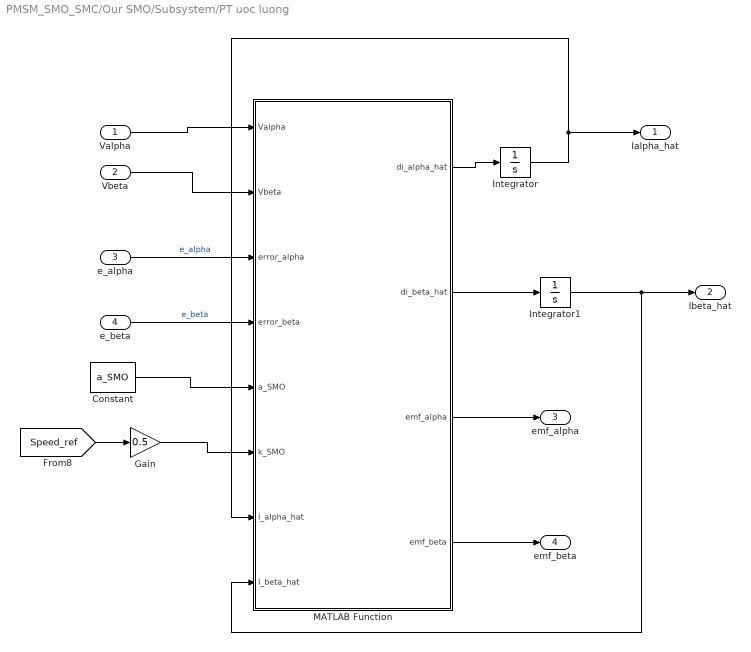
== system PMSM_SMO_SMC/Our SMO/Subsystem/PT uoc luong ==
  Valpha : Inport
  Vbeta : Inport  Port=2
  e_alpha : Inport  Port=3
  e_beta : Inport  Port=4
  Constant : Constant  Value=a_SMO
  Gain : Gain  Gain=0.5
  Integrator : Integrator
  Integrator1 : Integrator
  MATLAB Function : MATLAB Function  TreatAsAtomicUnit=on
  Ialpha_hat : Outport
  Ibeta_hat : Outport  Port=2
  emf_alpha : Outport  Port=3
  emf_beta : Outport  Port=4
  wires:
  Valpha/1 -> MATLAB Function/1(Valpha)
  Vbeta/1 -> MATLAB Function/2(Vbeta)
  e_alpha/1 -> MATLAB Function/3(error_alpha)  "e_alpha"
  e_beta/1 -> MATLAB Function/4(error_beta)  "e_beta"
  MATLAB Function/1(di_alpha_hat) -> Integrator/1
  MATLAB Function/2(di_beta_hat) -> Integrator1/1
  Integrator/1 -> MATLAB Function/7(I_alpha_hat), Ialpha_hat/1
  Integrator1/1 -> Ibeta_hat/1, MATLAB Function/8(I_beta_hat)
  MATLAB Function/4(emf_beta) -> emf_beta/1
  MATLAB Function/3(emf_alpha) -> emf_alpha/1
  Constant/1 -> MATLAB Function/5(a_SMO)
  Gain/1 -> MATLAB Function/6(k_SMO)
  [Speed_ref] -> Gain/1

== matlab function PMSM_SMO_SMC/Our SMO/Subsystem/PT uoc luong/MATLAB Function ==
  settings: updateMethod=DISCRETE  sampleTime=1E-4
  data: Valpha input; di_alpha_hat output; Vbeta input; error_alpha input; error_beta input; di_beta_hat output; emf_alpha output; emf_beta output; a_SMO input; k_SMO input; I_alpha_hat input; I_beta_hat input
function [di_alpha_hat, di_beta_hat, emf_alpha, emf_beta] = SMO_Observer(Valpha, Vbeta, error_alpha, error_beta, a_SMO,k_SMO, I_alpha_hat, I_beta_hat)
    Rs = 2.875; %Stator Resistance
    Ls = 8.5e-3; %Stator Inductance
    k = k_SMO ;
    a = a_SMO ;

    % Tính toán H_alpha và H_beta
    H_alpha = (2./(1 + exp(-a * error_alpha/20))) - 1;
    H_beta = (2./(1 + exp(-a * error_beta/20))) - 1;

    % Tính toán di_alpha_hat và di_beta_hat
    di_alpha_hat = -(Rs/Ls)*I_alpha_hat + (1/Ls)*Valpha - (1/Ls)*k*H_alpha;
    di_beta_hat = -(Rs/Ls)*I_beta_hat + (1/Ls)*Vbeta - (1/Ls)*k*H_beta;

    % Tính toán emf_alpha và emf_beta (EMF components)
    emf_alpha = k * H_alpha;
    emf_beta = k * H_beta;
end

== matlab function PMSM_SMO_SMC/SMC_Speed_Controller/RBF calculation a^/RBF ==
  data: e input; h1 output; h2 output; h3 output
function [h1,h2,h3] = Calculate_RBF(e)
theta = 0.36;
cij = [-1 0 1];
h1 = exp(-norm(e - cij(1))^2/theta);
h2 = exp(-norm(e - cij(2))^2/theta);
h3 = exp(-norm(e - cij(3))^2/theta);

== matlab function PMSM_SMO_SMC/FOC_PMSM/PMSM Model/MATLAB Function3 ==
  settings: updateMethod=DISCRETE  sampleTime=1E-4
  data: theta_hat input; omega_hat output
function omega_hat = CalculateOmega(theta_hat)
    % Khởi tạo biến persistent để lưu trữ giá trị theta_hat của bước trước
    persistent theta_hat_prev delta_theta;
    if isempty(theta_hat_prev)
        theta_hat_prev = theta_hat;
    end

    if isempty(delta_theta)
        delta_theta = 0;
    end
    % Thời gian lấy mẫu, điều chỉnh theo hệ thống thực tế của bạn
    Ts = 0.0001;
    
    if ( abs(theta_hat - theta_hat_prev)> (3.14/2) )
       
    else
         delta_theta = (theta_hat - theta_hat_prev);
    end 

    % Tính toán tốc độ điện áp ước lượng omega_hat

   % omega_hat = 9.5493 * (theta_hat - theta_hat_prev) / Ts;
    omega_hat = 9.5493 * delta_theta / Ts;

    % Cập nhật giá trị theta_hat_prev cho vòng lặp tiếp theo
    theta_hat_prev = theta_hat;
end

== matlab function PMSM_SMO_SMC/FOC_PMSM/PMSM Model/0 - 2pi ==
  data: theta input; theta_adjusted output
function theta_adjusted = AdjustTheta(theta)
    % Điều chỉnh giá trị góc để nằm trong khoảng [-pi, pi]
    theta_adjusted = mod(theta + pi, 2*pi) - pi;
end

== matlab function PMSM_SMO_SMC/Our SMO/MATLAB Function3 ==
  settings: updateMethod=DISCRETE  sampleTime=1E-4
  data: theta_hat input; omega_hat output
function omega_hat = CalculateOmega(theta_hat)
    % Khởi tạo biến persistent để lưu trữ giá trị theta_hat của bước trước
    persistent theta_hat_prev delta_theta;
    if isempty(theta_hat_prev)
        theta_hat_prev = theta_hat +0.00001;
    end

    if isempty(delta_theta)
        delta_theta = 0;
    end
    % Thời gian lấy mẫu, điều chỉnh theo hệ thống thực tế của bạn
    Ts = 0.0001;
    
    if ( abs(theta_hat - theta_hat_prev)> (3.14/2) )
       
    else
         delta_theta = (theta_hat - theta_hat_prev);
    end 

    % Tính toán tốc độ điện áp ước lượng omega_hat

   % omega_hat = 9.5493 * (theta_hat - theta_hat_prev) / Ts;
    omega_hat = 9.5493 * delta_theta / Ts; 
    %omega_hat = delta_theta/Ts;

    % Cập nhật giá trị theta_hat_prev cho vòng lặp tiếp theo
    theta_hat_prev = theta_hat;
end

== matlab function PMSM_SMO_SMC/FOC_PMSM/PMSM Model/MATLAB Function ==
  data: omega_r input; e_alpha output; theta input; e_beta output
function [e_alpha, e_beta] = CalculateEMF(omega_r, theta)
    % Tham số từ thông
    lambda_f = 0.175;

    % Tính toán e_alpha và e_beta
    e_alpha = -lambda_f * omega_r * sin(theta);
    e_beta = lambda_f * omega_r * cos(theta);
end

== matlab function PMSM_SMO_SMC/SMC_Speed_Controller/MATLAB Function ==
  data: a output; b output; J parameter; TL parameter; B parameter; p parameter; lambda parameter; x1 input
function [a,b] = Calculate_a_b(J, TL, B, p, lambda, x1)

a = (1/J)*(-TL-B*x1);
b = (1/J)*(3/2)*p*lambda;

== matlab function PMSM_SMO_SMC/SMC_Speed_Controller/SMC ==
  data: a input; u output; b input; y_ref_dot input; y input; s input; eq_s output
function [u,eq_s] = fcn(a,b,y_ref_dot,y,s)
%Parameter of eq_s_new
n = 2;
k = 1000;
m = 4;
del = 10;
ep = 1;
psi = 0.1;
% Tính toán hàm eq_s_new
eq_s_new = (k) / (ep + (1 + 1 / (abs(s/20)^m) - ep) * (1 + abs(s/20 + psi)^-n));
eq_s = k/(ep+(1+1/abs(s/400)-ep)*exp(-psi*abs(s/400)));
%eq_s = 10*abs(s);
u = (1/b)*(-a + y_ref_dot + eq_s*sat(s));

function y = sat(x)
    if(x > 1)
        y = 1;
    elseif (x < -1)
        y = -1;
    else
        y = x;
    end
